simulink model "gato_aspiradora"  (R2022b)
settings: Solver=FixedStepAuto  StartTime=0.0  StopTime=3  FixedStep=0.00001  RelTol=1e-3
settings Model: Creator=Fran  LastModifiedBy=Fran

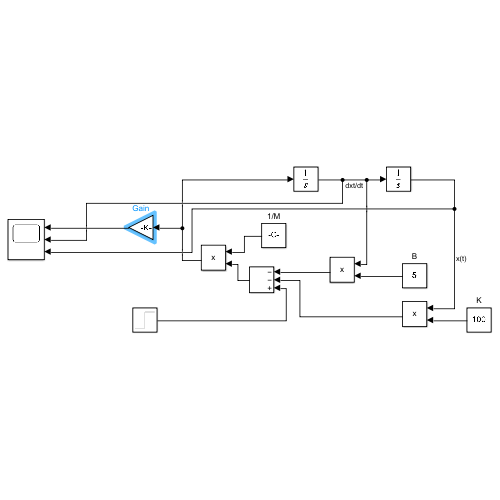
[thumbnail: Simulink's stored preview of the top-level diagram]
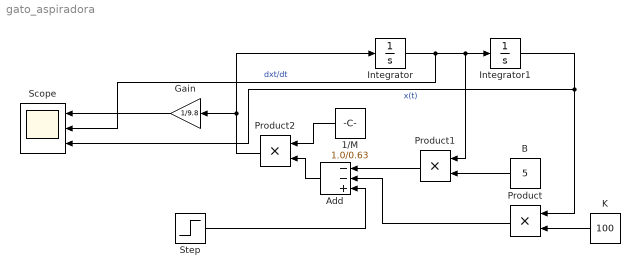
== system gato_aspiradora ==
  1/M : Constant  Value=1.0/0.63
  Add : Sum  Inputs=--+
  B : Constant  Value=5
  Gain : Gain  Gain=1/9.8
  Integrator : Integrator
  Integrator1 : Integrator
  K : Constant  Value=100
  Product : Product
  Product1 : Product
  Product2 : Product
  Scope : Scope  NumInputPorts=3
  Step : Step  Time=0  After=9.8 * 0.1  SampleTime=0
  wires:
  Integrator/1 -> Scope/2, Product1/1, Integrator1/1  "dxt/dt"
  Integrator1/1 -> Scope/3, Product/1  "x(t)"
  K/1 -> Product/2
  B/1 -> Product1/2
  Add/1 -> Product2/2
  1/M/1 -> Product2/1
  Product2/1 -> Gain/1, Integrator/1
  Product1/1 -> Add/1
  Product/1 -> Add/2
  Step/1 -> Add/3
  Gain/1 -> Scope/1
